simulink model "hardware_control"  (R2016b)
settings: Solver=FixedStepDiscrete  StartTime=0.0  StopTime=inf  FixedStep=elmo_sample_time  RelTol=1e-3
settings Model: ExplicitPartitioning=on  Creator=wmartin  LastModifiedBy=Will
settings SolverCC: EnableConcurrentExecution=on  ConcurrentTasks=on
settings DataIOCC: MaxDataPoints=1000000000  SaveFormat=StructureWithTime  SignalLogging=off  DSMLogging=off  VisualizeSimOutput=off
settings OptimizationCC: BlockReduction=off  OptimizeBlockIOStorage=off  BufferReuse=off  GlobalBufferReuse=off  ExpressionFolding=off  ExpressionDepthLimit=2147483647  LocalBlockOutputs=off  LifeSpan=inf  SimCompilerOptimization=on
settings DebuggingCC: UnderspecifiedInitializationDetection=Classic  MergeDetectMultiDrivingBlocksExec=none  SolverPrmCheckMsg=warning  StateNameClashWarn=warning  SFUnexpectedBacktrackingDiag=warning  SFNoUnconditionalDefaultTransitionDiag=warning  SFExecutionAtInitializationDiag=none
settings HardwareCC: ProdBitPerPointer=32  ProdBitPerSizeT=32  ProdBitPerPtrDiffT=32  ProdLargestAtomicFloat=None  ProdWordSize=32  ProdLongLongMode=on  ProdHWDeviceType=Generic->32-bit x86 compatible
settings ModelReferenceCC: UpdateModelReferenceTargets=IfOutOfDate  ModelReferenceNumInstancesAllowed=Single  ModelReferenceMinAlgLoopOccurrences=on  PropagateSignalLabelsOutOfModel=off
settings RTWCC: SystemTargetFile=slrt.tlc  TemplateMakefile=slrt_default_tmf  Description=Simulink Real-Time  RTWVerbose=off  RTWCompilerOptimization=on
settings CodeAppCC: MaxIdLength=256
settings SimulinkRealTimeCC: GeneratePreprocessorConditionals=Disable all  RL32LogBufSizeModifier=5e7
settings ConfigComp: CovMetricSettings=dw  CovHtmlReporting=on  CovSaveCumulativeToWorkspaceVar=on  CovSaveSingleToWorkspaceVar=on  CovExternalEMLEnable=off  CovSFcnEnable=off

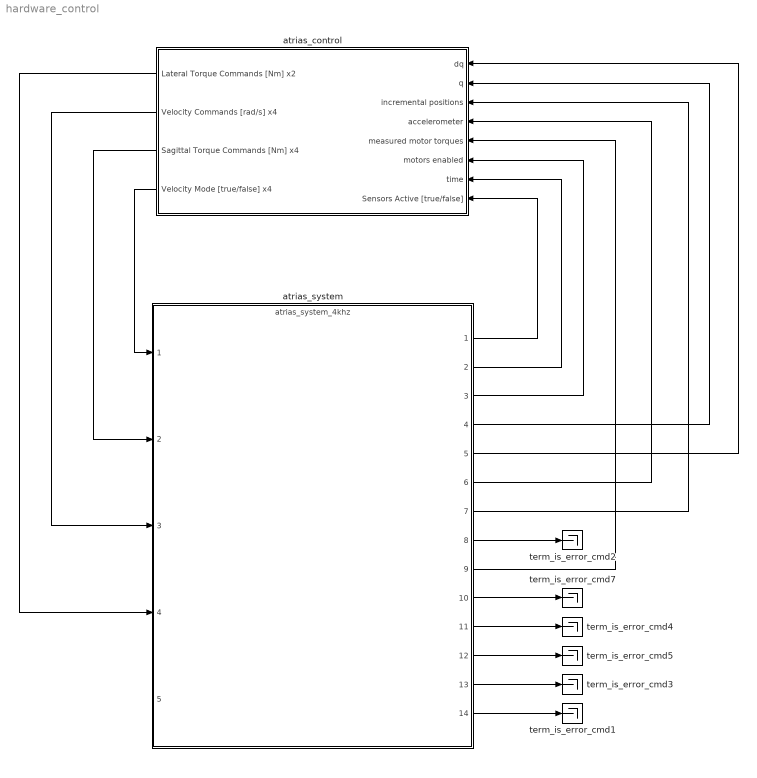
== system hardware_control ==
  atrias_control : Subsystem
  atrias_system : ModelReference  ModelNameDialog=atrias_system_4khz  SimulationMode=Normal  ModelReferenceVersion=1.3166
  term_is_error_cmd{1..5,7} (6 alike) : Terminator
  wires:
  atrias_system/2 -> atrias_control/7(time)
  atrias_system/9 -> atrias_control/5(measured motor torques)
  atrias_system/11 -> term_is_error_cmd4/1
  atrias_system/12 -> term_is_error_cmd5/1
  atrias_system/14 -> term_is_error_cmd1/1
  atrias_control/2(Velocity Commands [rad/s] x4) -> atrias_system/3
  atrias_system/3 -> atrias_control/6(motors enabled)
  atrias_control/1(Lateral Torque Commands [Nm] x2) -> atrias_system/4
  atrias_system/13 -> term_is_error_cmd3/1
  atrias_system/4 -> atrias_control/2(q)
  atrias_system/5 -> atrias_control/1(dq)
  atrias_control/4(Velocity Mode [true/false] x4) -> atrias_system/1
  atrias_control/3(Sagittal Torque Commands [Nm] x4) -> atrias_system/2
  atrias_system/6 -> atrias_control/4(accelerometer)
  atrias_system/1 -> atrias_control/8(Sensors Active [true/false])
  atrias_system/7 -> atrias_control/3(incremental positions)
  atrias_system/8 -> term_is_error_cmd2/1
  atrias_system/10 -> term_is_error_cmd7/1

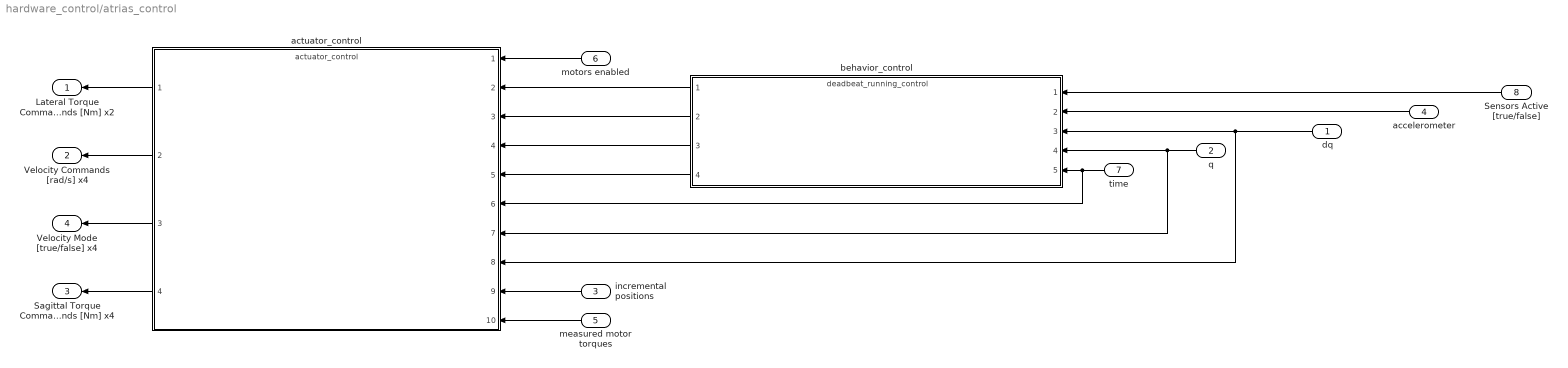
== system hardware_control/atrias_control ==
  dq : Inport  OutDataTypeStr=double  PortDimensions=13  SampleTime=[0.001,0]
  q : Inport  Port=2  OutDataTypeStr=double  PortDimensions=13  SampleTime=[0.001,0]
  incremental positions : Inport  Port=3  OutDataTypeStr=double  PortDimensions=4  SampleTime=[0.00025000000000000001,0]
  accelerometer : Inport  Port=4  OutDataTypeStr=double  PortDimensions=3  SampleTime=[0.001,0]
  measured motor torques : Inport  Port=5  OutDataTypeStr=double  PortDimensions=4  SampleTime=[0.00025000000000000001,0]
  motors enabled : Inport  Port=6  OutDataTypeStr=boolean  PortDimensions=1  SampleTime=[0.00025000000000000001,0]
  time : Inport  Port=7  OutDataTypeStr=double  PortDimensions=1  SampleTime=[0.00025000000000000001,0]
  Sensors Active [true/false] : Inport  Port=8  PortDimensions=1  SampleTime=[0.001,0]
  actuator_control : ModelReference  ModelNameDialog=actuator_control  SimulationMode=Normal  ModelReferenceVersion=1.1491
  behavior_control : ModelReference  ModelNameDialog=deadbeat_running_control  SimulationMode=Normal  ModelReferenceVersion=1.5053
  Lateral Torque Commands [Nm] x2 : Outport  OutDataTypeStr=double  PortDimensions=2  SampleTime=[0.00025000000000000001,0]  InitialOutput=[0 0]
  Velocity Commands [rad/s] x4 : Outport  Port=2  OutDataTypeStr=double  PortDimensions=4  SampleTime=[0.00025000000000000001,0]  InitialOutput=[0 0 0 0]
  Sagittal Torque Commands [Nm] x4 : Outport  Port=3  OutDataTypeStr=double  PortDimensions=4  SampleTime=[0.00025000000000000001,0]  InitialOutput=[0 0 0 0]
  Velocity Mode [true/false] x4 : Outport  Port=4  OutDataTypeStr=boolean  PortDimensions=4  SampleTime=[0.00025000000000000001,0]  InitialOutput=[true true true true]
  wires:
  motors enabled/1 -> actuator_control/1
  accelerometer/1 -> behavior_control/2
  actuator_control/1 -> Lateral Torque Commands [Nm] x2/1
  dq/1 -> actuator_control/8, behavior_control/3
  incremental positions/1 -> actuator_control/9
  measured motor torques/1 -> actuator_control/10
  behavior_control/1 -> actuator_control/2
  behavior_control/2 -> actuator_control/3
  q/1 -> actuator_control/7, behavior_control/4
  time/1 -> actuator_control/6, behavior_control/5
  Sensors Active [true/false]/1 -> behavior_control/1
  actuator_control/3 -> Velocity Mode [true/false] x4/1
  actuator_control/2 -> Velocity Commands [rad/s] x4/1
  actuator_control/4 -> Sagittal Torque Commands [Nm] x4/1
  behavior_control/4 -> actuator_control/5
  behavior_control/3 -> actuator_control/4
